simulink model "sslink"  (R2016a)
settings: Solver=VariableStepAuto  StartTime=0.0  StopTime=30  RelTol=1e-3
settings Model: Creator=user  LastModifiedBy=user

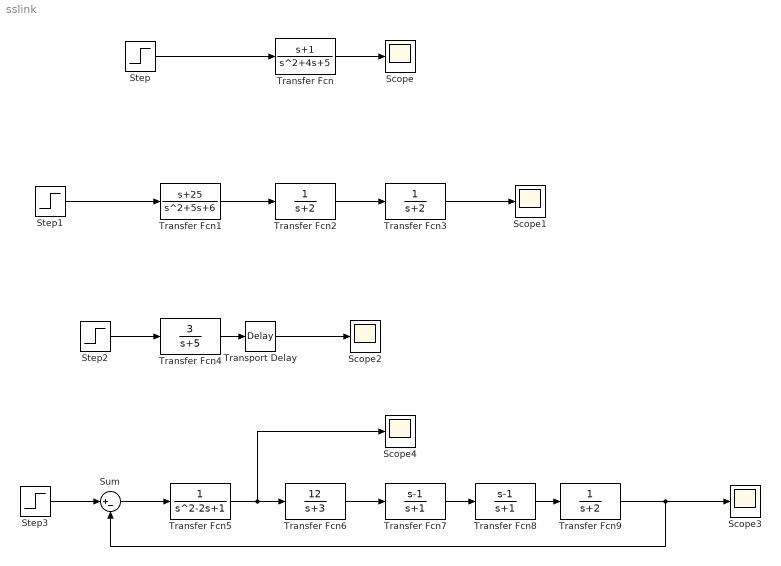
== system sslink ==
  Scope{,1..4} (5 alike) : Scope
  Step{,1..3} (4 alike) : Step  SampleTime=0
  Sum : Sum  Inputs=|+-
  Transfer Fcn : TransferFcn  Numerator=[1 1]  Denominator=[1 4 5]
  Transfer Fcn1 : TransferFcn  Numerator=[1 25]  Denominator=[1 5 6]
  Transfer Fcn2 : TransferFcn  Denominator=[1 2]
  Transfer Fcn3 : TransferFcn  Denominator=[1 2]
  Transfer Fcn4 : TransferFcn  Numerator=[3]  Denominator=[1 5]
  Transfer Fcn5 : TransferFcn  Denominator="[1 -2  1]"
  Transfer Fcn6 : TransferFcn  Numerator=[12]  Denominator=[1 3]
  Transfer Fcn7 : TransferFcn  Numerator=[1 -1]  Denominator=[1 1]
  Transfer Fcn8 : TransferFcn  Numerator=[1 -1]  Denominator=[1 1]
  Transfer Fcn9 : TransferFcn  Denominator=[1 2]
  Transport Delay : TransportDelay  DelayTime=0.5
  wires:
  Transfer Fcn/1 -> Scope/1
  Step/1 -> Transfer Fcn/1
  Transfer Fcn1/1 -> Transfer Fcn2/1
  Transfer Fcn2/1 -> Transfer Fcn3/1
  Transfer Fcn3/1 -> Scope1/1
  Step1/1 -> Transfer Fcn1/1
  Transfer Fcn4/1 -> Transport Delay/1
  Step2/1 -> Transfer Fcn4/1
  Transport Delay/1 -> Scope2/1
  Transfer Fcn5/1 -> Scope4/1, Transfer Fcn6/1
  Transfer Fcn6/1 -> Transfer Fcn7/1
  Transfer Fcn7/1 -> Transfer Fcn8/1
  Transfer Fcn8/1 -> Transfer Fcn9/1
  Transfer Fcn9/1 -> Sum/2, Scope3/1
  Step3/1 -> Sum/1
  Sum/1 -> Transfer Fcn5/1
